simulink model "sp2t_TestBed1_org"  (Simulink 10.0)
settings: Solver=FixedStepDiscrete  StartTime=0.0  StopTime=1  FixedStep=1  RelTol=1e-3  EnableMultiTasking=on
undefined symbols (not defined in the file): MWS
libraries: Lib_Thermo_SP2T_TMATS x1
settings Model: Creator=jwchapm2  LastModifiedBy=annonymous
settings DataIOCC: LimitDataPoints=on
settings OptimizationCC: ExpressionDepthLimit=2147483647
settings DebuggingCC: SolverPrmCheckMsg=warning  StateNameClashWarn=warning
settings GRTTargetCC: GeneratePreprocessorConditionals=Disable all  CombineOutputUpdateFcns=on  GRTInterface=off
settings ConfigComp: CovExternalEMLEnable=off

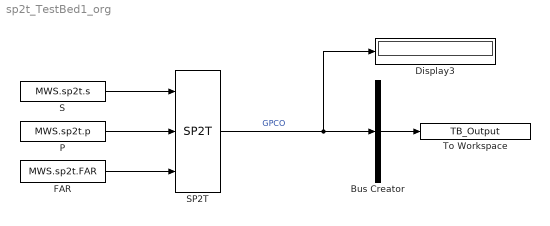
== system sp2t_TestBed1_org ==
  Bus Creator : BusCreator  Inputs=1
  Display3 : Display
  FAR : Constant  Value=MWS.sp2t.FAR
  P : Constant  Value=MWS.sp2t.p
  S : Constant  Value=MWS.sp2t.s
  SP2T : Lib_Thermo_SP2T_TMATS/SP2T
  To Workspace : ToWorkspace  VariableName=TB_Output  SampleTime=-1
  wires:
  FAR/1 -> SP2T/3
  SP2T/1 -> Display3/1, Bus Creator/1  "GPCO"
  Bus Creator/1 -> To Workspace/1
  P/1 -> SP2T/2
  S/1 -> SP2T/1
